simulink model "Md61Md62CalibSet"  (R2018b)
settings: Solver=FixedStepDiscrete  StartTime=0.0  StopTime=10.0  FixedStep=0.01  RelTol=1e-3
undefined symbols (not defined in the file or in its folder): KeSMSuFirstRwStBackPosDelta_Val, KeSMSuFirstRwStCushFoldPosDelta_Val, KeSMSuFirstRwStFwdBkwdPosDelta_Val, KeSMSuThrdRwCushFoldPosDelta_Val, KeSMSwAcsMd30PassStBkReclnUpwdDnwdPos1_Val, KeSMSwAcsMd30PassStBkReclnUpwdDnwdPos1Max_Val, KeSMSwAcsMd30PassStBkReclnUpwdDnwdPos1Min_Val, KeSMSwAcsMd30PassStFldUpwdDnwdPos1_Val, KeSMSwAcsMd30PassStFrwdBkwdPos1_Val, KeSMSwAcsMd30PassStFrwdBkwdPos1Max_Val, KeSMSwAcsMd30PassStFrwdBkwdPos1Min_Val, KeSMSwSeatBkLimitPos_Val, KeSMSwSeatBkLimitPosDelt_Val
libraries: StIsPosChkLib x2
(part 3 of 5)

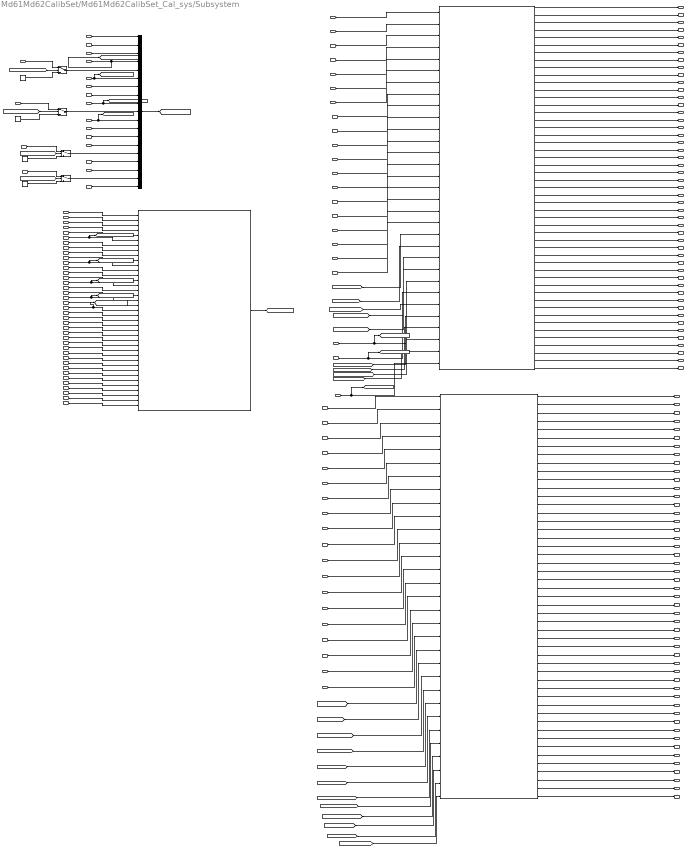
== system Md61Md62CalibSet/Md61Md62CalibSet_Cal_sys/Subsystem ==
  EepMd61PassStBkReclnTrgtPos_Val_read : Inport
  EepMd61PassStCshnFldTrgtPos_Val_read : Inport  Port=2
  EepMd61PassStFwdBkwdTrgtPos_Val_read : Inport  Port=3
  EepMd61SecRwLtStBkReclnTrgtPos_Val_read : Inport  Port=4
  EepMd61SecRwLtStCushFrntTrgtPos_Val_read : Inport  Port=5
  EepMd61SecRwLtStFwdBkwdTrgtPos_Val_read : Inport  Port=6
  EepMd61SecRwLtStLgrstInwdOtwdTrgtPos_Val_read : Inport  Port=7
  EepMd61SecRwLtStLgrstUpwdDnwdTrgtPos_Val_read : Inport  Port=8
  EepMd61SecRwRtStBkReclnTrgtPos_Val_read : Inport  Port=9
  EepMd61SecRwRtStCushFrntTrgtPos_Val_read : Inport  Port=10
  EepMd61SecRwRtStFwdBkwdTrgtPos_Val_read : Inport  Port=11
  EepMd61SecRwRtStLgrstInwdOtwdTrgtPos_Val_read : Inport  Port=12
  EepMd61SecRwRtStLgrstUpwdDnwdTrgtPos_Val_read : Inport  Port=13
  EepMd61ThdRwLtStBkReclnTrgtPos_Val_read : Inport  Port=14
  EepMd61ThdRwLtStCshnFldTrgtPos_Val_read : Inport  Port=15
  EepMd61ThdRwLtStFwdBkwdTrgtPos_Val_read : Inport  Port=16
  EepMd61ThdRwRtStBkReclnTrgtPos_Val_read : Inport  Port=17
  EepMd61ThdRwRtStCshnFldTrgtPos_Val_read : Inport  Port=18
  EepMd61ThdRwRtStFwdBkwdTrgtPos_Val_read : Inport  Port=19
  EepMd62PassStBkReclnTrgtPos_Val_read : Inport  Port=20
  EepMd62PassStCshnFldTrgtPos_Val_read : Inport  Port=21
  EepMd62PassStFwdBkwdTrgtPos_Val_read : Inport  Port=22
  EepMd62SecRwLtStBkReclnTrgtPos_Val_read : Inport  Port=23
  EepMd62SecRwLtStCushFrntTrgtPos_Val_read : Inport  Port=24
  EepMd62SecRwLtStFwdBkwdTrgtPos_Val_read : Inport  Port=25
  EepMd62SecRwLtStLgrstInwdOtwdTrgtPos_Val_read : Inport  Port=26
  EepMd62SecRwLtStLgrstUpwdDnwdTrgtPos_Val_read : Inport  Port=27
  EepMd62SecRwRtStBkReclnTrgtPos_Val_read : Inport  Port=28
  EepMd62SecRwRtStCushFrntTrgtPos_Val_read : Inport  Port=29
  EepMd62SecRwRtStFwdBkwdTrgtPos_Val_read : Inport  Port=30
  EepMd62SecRwRtStLgrstInwdOtwdTrgtPos_Val_read : Inport  Port=31
  EepMd62SecRwRtStLgrstUpwdDnwdTrgtPos_Val_read : Inport  Port=32
  EepMd62ThdRwLtStBkReclnTrgtPos_Val_read : Inport  Port=33
  EepMd62ThdRwLtStCshnFldTrgtPos_Val_read : Inport  Port=34
  EepMd62ThdRwLtStFwdBkwdTrgtPos_Val_read : Inport  Port=35
  EepMd62ThdRwRtStBkReclnTrgtPos_Val_read : Inport  Port=36
  EepMd62ThdRwRtStCshnFldTrgtPos_Val_read : Inport  Port=37
  EepMd62ThdRwRtStFwdBkwdTrgtPos_Val_read : Inport  Port=38
  IfVeSMSbPassStBkReclnUpwdDnwdMovConfig_Val_read : Inport  Port=39
  IfVeSMSbPassStFldUpwdDnwdMovConfig_Val_read : Inport  Port=40
  IfVeSMSbPassStFrwdBkwdMovConfig_Val_read : Inport  Port=41
  IfVeSMSbSecRwLtSLgrstExpdMovConfig_Val_read : Inport  Port=42
  IfVeSMSbSecRwLtStBkReclnUpwdDnwdMovConfig_Val_read : Inport  Port=43
  IfVeSMSbSecRwLtStCshnFrntUpwdDnwdMovConfig_Val_read : Inport  Port=44
  IfVeSMSbSecRwLtStFrwdBkwdMovConfig_Val_read : Inport  Port=45
  IfVeSMSbSecRwLtStLgrstUpwdMovConfig_Val_read : Inport  Port=46
  IfVeSMSbSecRwRtSLgrstExpdMovConfig_Val_read : Inport  Port=47
  IfVeSMSbSecRwRtStBkReclnUpwdDnwdMovConfig_Val_read : Inport  Port=48
  IfVeSMSbSecRwRtStCshnFrntUpwdDnwdMovConfig_Val_read : Inport  Port=49
  IfVeSMSbSecRwRtStFrwdBkwdMovConfig_Val_read : Inport  Port=50
  IfVeSMSbSecRwRtStLgrstUpwdMovConfig_Val_read : Inport  Port=51
  IfVeSMSbThdRwLtStBkReclnUpwdDnwdMovConfig_Val_read : Inport  Port=52
  IfVeSMSbThdRwLtStCshnFldUpwdDnwdMovConfig_Val_read : Inport  Port=53
  IfVeSMSbThdRwLtStFrwdBkwdMovConfig_Val_read : Inport  Port=54
  IfVeSMSbThdRwRtStBkReclnUpwdDnwdMovConfig_Val_read : Inport  Port=55
  IfVeSMSbThdRwRtStCshnFldUpwdDnwdMovConfig_Val_read : Inport  Port=56
  IfVeSMSbThdRwRtStFrwdBkwdMovConfig_Val_read : Inport  Port=57
  IfVeSMSuPassStBkReclnUpwdDnwdPos_Val_read : Inport  Port=58
  IfVeSMSuPassStBkReclnUpwdDnwdPosV_Val_read : Inport  Port=59
  IfVeSMSuPassStFldUpwdDnwdPos_Val_read : Inport  Port=60
  IfVeSMSuPassStFldUpwdDnwdPosV_Val_read : Inport  Port=61
  IfVeSMSuPassStFrwdBkwdPos_Val_read : Inport  Port=62
  IfVeSMSuPassStFrwdBkwdPosV_Val_read : Inport  Port=63
  IfVeSMSuSecRwLtStBkReclnUpwdDnwdPos_Val_read : Inport  Port=64
  IfVeSMSuSecRwLtStBkReclnUpwdDnwdPosV_Val_read : Inport  Port=65
  IfVeSMSuSecRwLtStFrwdBkwdPos_Val_read : Inport  Port=66
  IfVeSMSuSecRwLtStFrwdBkwdPosV_Val_read : Inport  Port=67
  IfVeSMSuSecRwLtStLgrstOtwdInwdPos_Val_read : Inport  Port=68
  IfVeSMSuSecRwLtStLgrstOtwdInwdPosV_Val_read : Inport  Port=69
  IfVeSMSuSecRwLtStLgrstUpwdDnwdPos_Val_read : Inport  Port=70
  IfVeSMSuSecRwLtStLgrstUpwdDnwdPosV_Val_read : Inport  Port=71
  IfVeSMSuSecRwLtStZeroPos_Val_read : Inport  Port=72
  IfVeSMSuSecRwLtStZeroPosV_Val_read : Inport  Port=73
  IfVeSMSuSecRwRtStBkReclnUpwdDnwdPos_Val_read : Inport  Port=74
  IfVeSMSuSecRwRtStBkReclnUpwdDnwdPosV_Val_read : Inport  Port=75
  IfVeSMSuSecRwRtStFrwdBkwdPos_Val_read : Inport  Port=76
  IfVeSMSuSecRwRtStFrwdBkwdPosV_Val_read : Inport  Port=77
  IfVeSMSuSecRwRtStLgrstOtwdInwdPos_Val_read : Inport  Port=78
  IfVeSMSuSecRwRtStLgrstOtwdInwdPosV_Val_read : Inport  Port=79
  IfVeSMSuSecRwRtStLgrstUpwdDnwdPos_Val_read : Inport  Port=80
  IfVeSMSuSecRwRtStLgrstUpwdDnwdPosV_Val_read : Inport  Port=81
  IfVeSMSuSecRwRtStZeroPos_Val_read : Inport  Port=82
  IfVeSMSuSecRwRtStZeroPosV_Val_read : Inport  Port=83
  IfVeSMSuThdRwLtStBkReclnUpwdDnwdPos_Val_read : Inport  Port=84
  IfVeSMSuThdRwLtStBkReclnUpwdDnwdPosV_Val_read : Inport  Port=85
  IfVeSMSuThdRwLtStCshnFldUpwdDnwdPos_Val_read : Inport  Port=86
  IfVeSMSuThdRwLtStCshnFldUpwdDnwdPosV_Val_read : Inport  Port=87
  IfVeSMSuThdRwLtStFrwdBkwdPos_Val_read : Inport  Port=88
  IfVeSMSuThdRwLtStFrwdBkwdPosV_Val_read : Inport  Port=89
  IfVeSMSuThdRwRtStBkReclnUpwdDnwdPos_Val_read : Inport  Port=90
  IfVeSMSuThdRwRtStBkReclnUpwdDnwdPosV_Val_read : Inport  Port=91
  IfVeSMSuThdRwRtStCshnFldUpwdDnwdPos_Val_read : Inport  Port=92
  IfVeSMSuThdRwRtStCshnFldUpwdDnwdPosV_Val_read : Inport  Port=93
  IfVeSMSuThdRwRtStFrwdBkwdPos_Val_read : Inport  Port=94
  IfVeSMSuThdRwRtStFrwdBkwdPosV_Val_read : Inport  Port=95
  StPassCmprtRestMdMemVirtCtrlReqMdadjust_Val_read : Inport  Port=96
  KeSMSwSeatBkLimitPos_Val : Inport  Port=97
  KeSMSwSeatBkLimitPosDelt_Val : Inport  Port=98
  modestate32_Val_read : Inport  Port=99
  Constant{,1..3} (4 alike) : Constant  Value=4095  OutDataTypeStr=uint16
  Md61Calib : Subsystem
  Md62Calib : Subsystem
  MemReqChk : Subsystem
  Mux : Mux  Inputs=19
  Switch{,1..3} (4 alike) : Switch  Criteria=u2 > Threshold
  Md61PassStBkReclnTrgtPos_Val_write : Outport
      settings: EnsureOutportIsVirtual=on
  Md61PassStBkReclnTrgtPosCalib_TrgtPosArray_write : Outport  Port=2
      settings: EnsureOutportIsVirtual=on
  Md61PassStCshnFldTrgtPosCalib_TrgtPosArray_write : Outport  Port=3
      settings: EnsureOutportIsVirtual=on
  Md61PassStFwdBkwdTrgtPosCalib_TrgtPosArray_write : Outport  Port=4
      settings: EnsureOutportIsVirtual=on
  Md61SecRwLtStBkReclnTrgtPosCalib_TrgtPosArray_write : Outport  Port=5
      settings: EnsureOutportIsVirtual=on
  Md61SecRwLtStCushFrntTrgtPosCalib_TrgtPosArray_write : Outport  Port=6
      settings: EnsureOutportIsVirtual=on
  Md61SecRwLtStFwdBkwdCalib_TrgtPosArray_write : Outport  Port=7
      settings: EnsureOutportIsVirtual=on
  Md61SecRwLtStLgrstInwdOtwdTrgtPosCalib_TrgtPosArray_write : Outport  Port=8
      settings: EnsureOutportIsVirtual=on
  Md61SecRwLtStLgrstUpwdDnwdTrgtPosCalib_TrgtPosArray_write : Outport  Port=9
      settings: EnsureOutportIsVirtual=on
  Md61ThdRwLtStBkReclnUpwdDnwdTrgtPosCalib_TrgtPosArray_write : Outport  Port=10
      settings: EnsureOutportIsVirtual=on
  Md61ThdRwLtStCshnFldUpwdDnwdTrgtPos_Val_write : Outport  Port=11
      settings: EnsureOutportIsVirtual=on
  Md61ThdRwLtStCshnFldUpwdDnwdTrgtPosCalib_TrgtPosArray_write : Outport  Port=12
      settings: EnsureOutportIsVirtual=on
  Md61ThdRwLtStFrwdBkwdPosTrgtPosCalib_TrgtPosArray_write : Outport  Port=13
      settings: EnsureOutportIsVirtual=on
  Md61ThdRwRtStCshnFldUpwdDnwdTrgtPos_Val_write : Outport  Port=14
      settings: EnsureOutportIsVirtual=on
  Md62PassStBkReclnTrgtPos_Val_write : Outport  Port=15
      settings: EnsureOutportIsVirtual=on
  Md62PassStBkReclnTrgtPosCalib_TrgtPosArray_write : Outport  Port=16
      settings: EnsureOutportIsVirtual=on
  Md62PassStCshnFldTrgtPosCalib_TrgtPosArray_write : Outport  Port=17
      settings: EnsureOutportIsVirtual=on
  Md62PassStFwdBkwdTrgtPosCalib_TrgtPosArray_write : Outport  Port=18
      settings: EnsureOutportIsVirtual=on
  Md62SecRwLtStBkReclnTrgtPosCalib_TrgtPosArray_write : Outport  Port=19
      settings: EnsureOutportIsVirtual=on
  Md62SecRwLtStCushFrntTrgtPosCalib_TrgtPosArray_write : Outport  Port=20
      settings: EnsureOutportIsVirtual=on
  Md62SecRwLtStFwdBkwdCalib_TrgtPosArray_write : Outport  Port=21
      settings: EnsureOutportIsVirtual=on
  Md62SecRwLtStLgrstInwdOtwdTrgtPosCalib_TrgtPosArray_write : Outport  Port=22
      settings: EnsureOutportIsVirtual=on
  Md62SecRwLtStLgrstUpwdDnwdTrgtPosCalib_TrgtPosArray_write : Outport  Port=23
      settings: EnsureOutportIsVirtual=on
  Md62ThdRwLtStBkReclnUpwdDnwdTrgtPosCalib_TrgtPosArray_write : Outport  Port=24
      settings: EnsureOutportIsVirtual=on
  Md62ThdRwLtStCshnFldUpwdDnwdTrgtPos_Val_write : Outport  Port=25
      settings: EnsureOutportIsVirtual=on
  Md62ThdRwLtStCshnFldUpwdDnwdTrgtPosCalib_TrgtPosArray_write : Outport  Port=26
      settings: EnsureOutportIsVirtual=on
  Md62ThdRwLtStFrwdBkwdPosTrgtPosCalib_TrgtPosArray_write : Outport  Port=27
      settings: EnsureOutportIsVirtual=on
  Md62ThdRwRtStCshnFldUpwdDnwdTrgtPos_Val_write : Outport  Port=28
      settings: EnsureOutportIsVirtual=on
  Md61SecRwRtStBkReclnTrgtPosCalib_TrgtPosArray_write : Outport  Port=29
      settings: EnsureOutportIsVirtual=on
  Md61SecRwRtStCushFrntTrgtPosCalib_TrgtPosArray_write : Outport  Port=30
      settings: EnsureOutportIsVirtual=on
  Md61SecRwRtStFwdBkwdCalib_TrgtPosArray_write : Outport  Port=31
      settings: EnsureOutportIsVirtual=on
  Md61SecRwRtStLgrstInwdOtwdTrgtPosCalib_TrgtPosArray_write : Outport  Port=32
      settings: EnsureOutportIsVirtual=on
  Md61SecRwRtStLgrstUpwdDnwdTrgtPosCalib_TrgtPosArray_write : Outport  Port=33
      settings: EnsureOutportIsVirtual=on
  Md61ThdRwRtStBkReclnUpwdDnwdTrgtPosCalib_TrgtPosArray_write : Outport  Port=34
      settings: EnsureOutportIsVirtual=on
  Md61ThdRwRtStCshnFldUpwdDnwdTrgtPosCalib_TrgtPosArray_write : Outport  Port=35
      settings: EnsureOutportIsVirtual=on
  Md61ThdRwRtStFrwdBkwdPosTrgtPosCalib_TrgtPosArray_write : Outport  Port=36
      settings: EnsureOutportIsVirtual=on
  Md62SecRwRtStBkReclnTrgtPosCalib_TrgtPosArray_write : Outport  Port=37
      settings: EnsureOutportIsVirtual=on
  Md62SecRwRtStCushFrntTrgtPosCalib_TrgtPosArray_write : Outport  Port=38
      settings: EnsureOutportIsVirtual=on
  Md62SecRwRtStFwdBkwdCalib_TrgtPosArray_write : Outport  Port=39
      settings: EnsureOutportIsVirtual=on
  Md62SecRwRtStLgrstInwdOtwdTrgtPosCalib_TrgtPosArray_write : Outport  Port=40
      settings: EnsureOutportIsVirtual=on
  Md62SecRwRtStLgrstUpwdDnwdTrgtPosCalib_TrgtPosArray_write : Outport  Port=41
      settings: EnsureOutportIsVirtual=on
  Md62ThdRwRtStBkReclnUpwdDnwdTrgtPosCalib_TrgtPosArray_write : Outport  Port=42
      settings: EnsureOutportIsVirtual=on
  Md62ThdRwRtStCshnFldUpwdDnwdTrgtPosCalib_TrgtPosArray_write : Outport  Port=43
      settings: EnsureOutportIsVirtual=on
  Md62ThdRwRtStFrwdBkwdPosTrgtPosCalib_TrgtPosArray_write : Outport  Port=44
      settings: EnsureOutportIsVirtual=on
  Md61PassStNeedFldOpn_Val_write : Outport  Port=45
      settings: EnsureOutportIsVirtual=on
  Md61PassStTrgtIsFld_Val_write : Outport  Port=46
      settings: EnsureOutportIsVirtual=on
  Md61ThdRwLtStNeedFldOpn_Val_write : Outport  Port=47
      settings: EnsureOutportIsVirtual=on
  Md61ThdRwLtStTrgtIsFld_Val_write : Outport  Port=48
      settings: EnsureOutportIsVirtual=on
  Md61ThdRwRtStNeedFldOpn_Val_write : Outport  Port=49
      settings: EnsureOutportIsVirtual=on
  Md61ThdRwRtStTrgtIsFld_Val_write : Outport  Port=50
      settings: EnsureOutportIsVirtual=on
  Md62PassStNeedFldOpn_Val_write : Outport  Port=51
      settings: EnsureOutportIsVirtual=on
  Md62PassStTrgtIsFld_Val_write : Outport  Port=52
      settings: EnsureOutportIsVirtual=on
  Md62ThdRwLtStNeedFldOpn_Val_write : Outport  Port=53
      settings: EnsureOutportIsVirtual=on
  Md62ThdRwLtStTrgtIsFld_Val_write : Outport  Port=54
      settings: EnsureOutportIsVirtual=on
  Md62ThdRwRtStNeedFldOpn_Val_write : Outport  Port=55
      settings: EnsureOutportIsVirtual=on
  Md62ThdRwRtStTrgtIsFld_Val_write : Outport  Port=56
      settings: EnsureOutportIsVirtual=on
  EepMd61PassStBkReclnTrgtPos_S_Val_write : Outport  Port=57
      settings: EnsureOutportIsVirtual=on
  EepMd61PassStCshnFldTrgtPos_S_Val_write : Outport  Port=58
      settings: EnsureOutportIsVirtual=on
  EepMd61PassStFwdBkwdTrgtPos_S_Val_write : Outport  Port=59
      settings: EnsureOutportIsVirtual=on
  EepMd61SecRwLtStBkReclnTrgtPos_S_Val_write : Outport  Port=60
      settings: EnsureOutportIsVirtual=on
  EepMd61SecRwLtStCushFrntTrgtPos_S_Val_write : Outport  Port=61
      settings: EnsureOutportIsVirtual=on
  EepMd61SecRwLtStFwdBkwdTrgtPos_S_Val_write : Outport  Port=62
      settings: EnsureOutportIsVirtual=on
  EepMd61SecRwLtStLgrstInwdOtwdTrgtPos_S_Val_write : Outport  Port=63
      settings: EnsureOutportIsVirtual=on
  EepMd61SecRwLtStLgrstUpwdDnwdTrgtPos_S_Val_write : Outport  Port=64
      settings: EnsureOutportIsVirtual=on
  EepMd61SecRwRtStBkReclnTrgtPos_S_Val_write : Outport  Port=65
      settings: EnsureOutportIsVirtual=on
  EepMd61SecRwRtStCushFrntTrgtPos_S_Val_write : Outport  Port=66
      settings: EnsureOutportIsVirtual=on
  EepMd61SecRwRtStFwdBkwdTrgtPos_S_Val_write : Outport  Port=67
      settings: EnsureOutportIsVirtual=on
  EepMd61SecRwRtStLgrstInwdOtwdTrgtPos_S_Val_write : Outport  Port=68
      settings: EnsureOutportIsVirtual=on
  EepMd61SecRwRtStLgrstUpwdDnwdTrgtPos_S_Val_write : Outport  Port=69
      settings: EnsureOutportIsVirtual=on
  EepMd61ThdRwLtStBkReclnTrgtPos_S_Val_write : Outport  Port=70
      settings: EnsureOutportIsVirtual=on
  EepMd61ThdRwLtStCshnFldTrgtPos_S_Val_write : Outport  Port=71
      settings: EnsureOutportIsVirtual=on
  EepMd61ThdRwLtStFwdBkwdTrgtPos_S_Val_write : Outport  Port=72
      settings: EnsureOutportIsVirtual=on
  EepMd61ThdRwRtStBkReclnTrgtPos_S_Val_write : Outport  Port=73
      settings: EnsureOutportIsVirtual=on
  EepMd61ThdRwRtStCshnFldTrgtPos_S_Val_write : Outport  Port=74
      settings: EnsureOutportIsVirtual=on
  EepMd61ThdRwRtStFwdBkwdTrgtPos_S_Val_write : Outport  Port=75
      settings: EnsureOutportIsVirtual=on
  EepMd62PassStBkReclnTrgtPos_S_Val_write : Outport  Port=76
      settings: EnsureOutportIsVirtual=on
  EepMd62PassStCshnFldTrgtPos_S_Val_write : Outport  Port=77
      settings: EnsureOutportIsVirtual=on
  EepMd62PassStFwdBkwdTrgtPos_S_Val_write : Outport  Port=78
      settings: EnsureOutportIsVirtual=on
  EepMd62SecRwLtStBkReclnTrgtPos_S_Val_write : Outport  Port=79
      settings: EnsureOutportIsVirtual=on
  EepMd62SecRwLtStCushFrntTrgtPos_S_Val_write : Outport  Port=80
      settings: EnsureOutportIsVirtual=on
  EepMd62SecRwLtStFwdBkwdTrgtPos_S_Val_write : Outport  Port=81
      settings: EnsureOutportIsVirtual=on
  EepMd62SecRwLtStLgrstInwdOtwdTrgtPos_S_Val_write : Outport  Port=82
      settings: EnsureOutportIsVirtual=on
  EepMd62SecRwLtStLgrstUpwdDnwdTrgtPos_S_Val_write : Outport  Port=83
      settings: EnsureOutportIsVirtual=on
  EepMd62SecRwRtStBkReclnTrgtPos_S_Val_write : Outport  Port=84
      settings: EnsureOutportIsVirtual=on
  EepMd62SecRwRtStCushFrntTrgtPos_S_Val_write : Outport  Port=85
      settings: EnsureOutportIsVirtual=on
  EepMd62SecRwRtStFwdBkwdTrgtPos_S_Val_write : Outport  Port=86
      settings: EnsureOutportIsVirtual=on
  EepMd62SecRwRtStLgrstInwdOtwdTrgtPos_S_Val_write : Outport  Port=87
      settings: EnsureOutportIsVirtual=on
  EepMd62SecRwRtStLgrstUpwdDnwdTrgtPos_S_Val_write : Outport  Port=88
      settings: EnsureOutportIsVirtual=on
  EepMd62ThdRwLtStBkReclnTrgtPos_S_Val_write : Outport  Port=89
      settings: EnsureOutportIsVirtual=on
  EepMd62ThdRwLtStCshnFldTrgtPos_S_Val_write : Outport  Port=90
      settings: EnsureOutportIsVirtual=on
  EepMd62ThdRwLtStFwdBkwdTrgtPos_S_Val_write : Outport  Port=91
      settings: EnsureOutportIsVirtual=on
  EepMd62ThdRwRtStBkReclnTrgtPos_S_Val_write : Outport  Port=92
      settings: EnsureOutportIsVirtual=on
  EepMd62ThdRwRtStCshnFldTrgtPos_S_Val_write : Outport  Port=93
      settings: EnsureOutportIsVirtual=on
  EepMd62ThdRwRtStFwdBkwdTrgtPos_S_Val_write : Outport  Port=94
      settings: EnsureOutportIsVirtual=on
  Md61MemReq_Val_write : Outport  Port=95
      settings: EnsureOutportIsVirtual=on
  Md62MemReq_Val_write : Outport  Port=96
      settings: EnsureOutportIsVirtual=on
  Md61NotMem_Val_write : Outport  Port=97
      settings: EnsureOutportIsVirtual=on
  Md62NotMem_Val_write : Outport  Port=98
      settings: EnsureOutportIsVirtual=on
  wires:
  [MemReq] -> Md61Calib/21(MemReq)
  EepMd61PassStCshnFldTrgtPos_Val_read/1 -> Md61Calib/2(EepMd61PassStCshnFldTrgtPos_Val_read)
  EepMd61PassStBkReclnTrgtPos_Val_read/1 -> Md61Calib/1(EepMd61PassStBkReclnTrgtPos_Val_read)
  EepMd61PassStFwdBkwdTrgtPos_Val_read/1 -> Md61Calib/3(EepMd61PassStFwdBkwdTrgtPos_Val_read)
  EepMd61SecRwLtStBkReclnTrgtPos_Val_read/1 -> Md61Calib/4(EepMd61SecRwLtStBkReclnTrgtPos_Val_read)
  EepMd61SecRwLtStCushFrntTrgtPos_Val_read/1 -> Md61Calib/5(EepMd61SecRwLtStCushFrntTrgtPos_Val_read)
  EepMd61SecRwLtStFwdBkwdTrgtPos_Val_read/1 -> Md61Calib/6(EepMd61SecRwLtStFwdBkwdTrgtPos_Val_read)
  EepMd61SecRwLtStLgrstInwdOtwdTrgtPos_Val_read/1 -> Md61Calib/7(EepMd61SecRwLtStLgrstInwdOtwdTrgtPos_Val_read)
  EepMd61SecRwLtStLgrstUpwdDnwdTrgtPos_Val_read/1 -> Md61Calib/8(EepMd61SecRwLtStLgrstUpwdDnwdTrgtPos_Val_read)
  EepMd61SecRwRtStBkReclnTrgtPos_Val_read/1 -> Md61Calib/9(EepMd61SecRwRtStBkReclnTrgtPos_Val_read)
  EepMd61SecRwRtStCushFrntTrgtPos_Val_read/1 -> Md61Calib/10(EepMd61SecRwRtStCushFrntTrgtPos_Val_read)
  EepMd61SecRwRtStFwdBkwdTrgtPos_Val_read/1 -> Md61Calib/11(EepMd61SecRwRtStFwdBkwdTrgtPos_Val_read)
  EepMd61SecRwRtStLgrstInwdOtwdTrgtPos_Val_read/1 -> Md61Calib/12(EepMd61SecRwRtStLgrstInwdOtwdTrgtPos_Val_read)
  EepMd61SecRwRtStLgrstUpwdDnwdTrgtPos_Val_read/1 -> Md61Calib/13(EepMd61SecRwRtStLgrstUpwdDnwdTrgtPos_Val_read)
  EepMd61ThdRwLtStBkReclnTrgtPos_Val_read/1 -> Md61Calib/14(EepMd61ThdRwLtStBkReclnTrgtPos_Val_read)
  EepMd61ThdRwLtStCshnFldTrgtPos_Val_read/1 -> Md61Calib/15(EepMd61ThdRwLtStCshnFldTrgtPos_Val_read)
  EepMd61ThdRwLtStFwdBkwdTrgtPos_Val_read/1 -> Md61Calib/16(EepMd61ThdRwLtStFwdBkwdTrgtPos_Val_read)
  EepMd61ThdRwRtStBkReclnTrgtPos_Val_read/1 -> Md61Calib/17(EepMd61ThdRwRtStBkReclnTrgtPos_Val_read)
  EepMd61ThdRwRtStCshnFldTrgtPos_Val_read/1 -> Md61Calib/18(EepMd61ThdRwRtStCshnFldTrgtPos_Val_read)
  EepMd61ThdRwRtStFwdBkwdTrgtPos_Val_read/1 -> Md61Calib/19(EepMd61ThdRwRtStFwdBkwdTrgtPos_Val_read)
  IfVeSMSbPassStBkReclnUpwdDnwdMovConfig_Val_read/1 -> MemReqChk/1(IfVeSMSbPassStBkReclnUpwdDnwdMovConfig_Val_read)
  IfVeSMSbPassStFldUpwdDnwdMovConfig_Val_read/1 -> MemReqChk/2(IfVeSMSbPassStFldUpwdDnwdMovConfig_Val_read)
  IfVeSMSbPassStFrwdBkwdMovConfig_Val_read/1 -> MemReqChk/3(IfVeSMSbPassStFrwdBkwdMovConfig_Val_read)
  IfVeSMSbSecRwLtSLgrstExpdMovConfig_Val_read/1 -> MemReqChk/4(IfVeSMSbSecRwLtSLgrstExpdMovConfig_Val_read)
  IfVeSMSbSecRwLtStBkReclnUpwdDnwdMovConfig_Val_read/1 -> MemReqChk/5(IfVeSMSbSecRwLtStBkReclnUpwdDnwdMovConfig_Val_read)
  IfVeSMSbSecRwLtStCshnFrntUpwdDnwdMovConfig_Val_read/1 -> [SecRwLtStCshnFrntUpwdDnwdMovConfig], MemReqChk/6(IfVeSMSbSecRwLtStCshnFrntUpwdDnwdMovConfig_Val_read)
  IfVeSMSbSecRwLtStFrwdBkwdMovConfig_Val_read/1 -> MemReqChk/7(IfVeSMSbSecRwLtStFrwdBkwdMovConfig_Val_read)
  IfVeSMSbSecRwLtStLgrstUpwdMovConfig_Val_read/1 -> MemReqChk/8(IfVeSMSbSecRwLtStLgrstUpwdMovConfig_Val_read)
  IfVeSMSbSecRwRtSLgrstExpdMovConfig_Val_read/1 -> MemReqChk/9(IfVeSMSbSecRwRtSLgrstExpdMovConfig_Val_read)
  IfVeSMSbSecRwRtStBkReclnUpwdDnwdMovConfig_Val_read/1 -> MemReqChk/10(IfVeSMSbSecRwRtStBkReclnUpwdDnwdMovConfig_Val_read)
  IfVeSMSbSecRwRtStCshnFrntUpwdDnwdMovConfig_Val_read/1 -> MemReqChk/11(IfVeSMSbSecRwRtStCshnFrntUpwdDnwdMovConfig_Val_read), [SecRwRtStCshnFrntUpwdDnwdMovConfig]
  IfVeSMSbSecRwRtStFrwdBkwdMovConfig_Val_read/1 -> MemReqChk/12(IfVeSMSbSecRwRtStFrwdBkwdMovConfig_Val_read)
  IfVeSMSbSecRwRtStLgrstUpwdMovConfig_Val_read/1 -> MemReqChk/13(IfVeSMSbSecRwRtStLgrstUpwdMovConfig_Val_read)
  IfVeSMSbThdRwLtStBkReclnUpwdDnwdMovConfig_Val_read/1 -> MemReqChk/14(IfVeSMSbThdRwLtStBkReclnUpwdDnwdMovConfig_Val_read)
  IfVeSMSbThdRwLtStCshnFldUpwdDnwdMovConfig_Val_read/1 -> [ThdRwLtStCshnFldUpwdDnwdMovConfig], MemReqChk/15(IfVeSMSbThdRwLtStCshnFldUpwdDnwdMovConfig_Val_read)
  IfVeSMSbThdRwLtStFrwdBkwdMovConfig_Val_read/1 -> MemReqChk/16(IfVeSMSbThdRwLtStFrwdBkwdMovConfig_Val_read)
  IfVeSMSbThdRwRtStBkReclnUpwdDnwdMovConfig_Val_read/1 -> MemReqChk/17(IfVeSMSbThdRwRtStBkReclnUpwdDnwdMovConfig_Val_read)
  IfVeSMSbThdRwRtStCshnFldUpwdDnwdMovConfig_Val_read/1 -> [ThdRwRtStCshnFldUpwdDnwdMovConfig], MemReqChk/18(IfVeSMSbThdRwRtStCshnFldUpwdDnwdMovConfig_Val_read)
  IfVeSMSbThdRwRtStFrwdBkwdMovConfig_Val_read/1 -> MemReqChk/19(IfVeSMSbThdRwRtStFrwdBkwdMovConfig_Val_read)
  IfVeSMSuPassStBkReclnUpwdDnwdPosV_Val_read/1 -> [IfVeSMSuPassStBkReclnUpwdDnwdPosV], MemReqChk/20(IfVeSMSuPassStBkReclnUpwdDnwdPosV_Val_read)
  IfVeSMSuPassStFldUpwdDnwdPosV_Val_read/1 -> MemReqChk/21(IfVeSMSuPassStFldUpwdDnwdPosV_Val_read)
  IfVeSMSuPassStFrwdBkwdPosV_Val_read/1 -> MemReqChk/22(IfVeSMSuPassStFrwdBkwdPosV_Val_read)
  IfVeSMSuSecRwLtStBkReclnUpwdDnwdPosV_Val_read/1 -> MemReqChk/23(IfVeSMSuSecRwLtStBkReclnUpwdDnwdPosV_Val_read)
  IfVeSMSuSecRwLtStFrwdBkwdPosV_Val_read/1 -> MemReqChk/24(IfVeSMSuSecRwLtStFrwdBkwdPosV_Val_read)
  IfVeSMSuSecRwLtStLgrstOtwdInwdPosV_Val_read/1 -> MemReqChk/25(IfVeSMSuSecRwLtStLgrstOtwdInwdPosV_Val_read)
  IfVeSMSuSecRwLtStLgrstUpwdDnwdPosV_Val_read/1 -> MemReqChk/26(IfVeSMSuSecRwLtStLgrstUpwdDnwdPosV_Val_read)
  IfVeSMSuSecRwLtStZeroPosV_Val_read/1 -> MemReqChk/27(IfVeSMSuSecRwLtStZeroPosV_Val_read)
  IfVeSMSuSecRwRtStBkReclnUpwdDnwdPosV_Val_read/1 -> MemReqChk/28(IfVeSMSuSecRwRtStBkReclnUpwdDnwdPosV_Val_read)
  IfVeSMSuSecRwRtStFrwdBkwdPosV_Val_read/1 -> MemReqChk/29(IfVeSMSuSecRwRtStFrwdBkwdPosV_Val_read)
  IfVeSMSuSecRwRtStLgrstOtwdInwdPosV_Val_read/1 -> MemReqChk/30(IfVeSMSuSecRwRtStLgrstOtwdInwdPosV_Val_read)
  IfVeSMSuSecRwRtStLgrstUpwdDnwdPosV_Val_read/1 -> MemReqChk/31(IfVeSMSuSecRwRtStLgrstUpwdDnwdPosV_Val_read)
  IfVeSMSuSecRwRtStZeroPosV_Val_read/1 -> MemReqChk/32(IfVeSMSuSecRwRtStZeroPosV_Val_read)
  IfVeSMSuThdRwLtStBkReclnUpwdDnwdPosV_Val_read/1 -> MemReqChk/33(IfVeSMSuThdRwLtStBkReclnUpwdDnwdPosV_Val_read)
  IfVeSMSuThdRwLtStCshnFldUpwdDnwdPosV_Val_read/1 -> MemReqChk/34(IfVeSMSuThdRwLtStCshnFldUpwdDnwdPosV_Val_read)
  IfVeSMSuThdRwLtStFrwdBkwdPosV_Val_read/1 -> MemReqChk/35(IfVeSMSuThdRwLtStFrwdBkwdPosV_Val_read)
  IfVeSMSuThdRwRtStBkReclnUpwdDnwdPosV_Val_read/1 -> MemReqChk/36(IfVeSMSuThdRwRtStBkReclnUpwdDnwdPosV_Val_read)
  IfVeSMSuThdRwRtStCshnFldUpwdDnwdPosV_Val_read/1 -> MemReqChk/37(IfVeSMSuThdRwRtStCshnFldUpwdDnwdPosV_Val_read)
  IfVeSMSuThdRwRtStFrwdBkwdPosV_Val_read/1 -> MemReqChk/38(IfVeSMSuThdRwRtStFrwdBkwdPosV_Val_read)
  StPassCmprtRestMdMemVirtCtrlReqMdadjust_Val_read/1 -> MemReqChk/39(StPassCmprtRestMdMemVirtCtrlReqMdadjust_Val_read)
  IfVeSMSuPassStBkReclnUpwdDnwdPos_Val_read/1 -> Mux/1
  IfVeSMSuPassStFldUpwdDnwdPos_Val_read/1 -> Mux/2
  IfVeSMSuPassStFrwdBkwdPos_Val_read/1 -> Mux/3
  IfVeSMSuSecRwLtStBkReclnUpwdDnwdPos_Val_read/1 -> Mux/4, [IfVeSMSuSecRwLtStBkReclnUpwdDnwdPos]
  IfVeSMSuSecRwRtStBkReclnUpwdDnwdPos_Val_read/1 -> [IfVeSMSuSecRwRtStBkReclnUpwdDnwdPos], Mux/9
  IfVeSMSuThdRwLtStBkReclnUpwdDnwdPos_Val_read/1 -> Mux/14
  IfVeSMSuThdRwLtStFrwdBkwdPos_Val_read/1 -> Mux/16
  IfVeSMSuThdRwRtStBkReclnUpwdDnwdPos_Val_read/1 -> Mux/17
  IfVeSMSuThdRwRtStFrwdBkwdPos_Val_read/1 -> Mux/19
  IfVeSMSuSecRwLtStFrwdBkwdPos_Val_read/1 -> [IfVeSMSuSecRwLtStFrwdBkwdPos], Mux/6
  IfVeSMSuSecRwLtStLgrstOtwdInwdPos_Val_read/1 -> Mux/7
  IfVeSMSuSecRwLtStLgrstUpwdDnwdPos_Val_read/1 -> Mux/8
  IfVeSMSuSecRwRtStFrwdBkwdPos_Val_read/1 -> [IfVeSMSuSecRwRtStFrwdBkwdPos], Mux/11
  IfVeSMSuSecRwRtStLgrstOtwdInwdPos_Val_read/1 -> Mux/12
  IfVeSMSuSecRwRtStLgrstUpwdDnwdPos_Val_read/1 -> Mux/13
  Mux/1 -> [CurrentPosArray]
  [CurrentPosArray] -> Md61Calib/20(CurrentPosArray)
  MemReqChk/1(MemReq) -> [MemReq]
  Md61Calib/2(Md61PassStBkReclnTrgtPosCalib_TrgtPosArray_write) -> Md61PassStBkReclnTrgtPosCalib_TrgtPosArray_write/1
  Md61Calib/3(Md61PassStCshnFldTrgtPosCalib_TrgtPosArray_write) -> Md61PassStCshnFldTrgtPosCalib_TrgtPosArray_write/1
  Md61Calib/1(Md61PassStBkReclnTrgtPos_Val_write) -> Md61PassStBkReclnTrgtPos_Val_write/1
  Md61Calib/4(Md61PassStFwdBkwdTrgtPosCalib_TrgtPosArray_write) -> Md61PassStFwdBkwdTrgtPosCalib_TrgtPosArray_write/1
  Md61Calib/5(Md61SecRwLtStBkReclnTrgtPosCalib_TrgtPosArray_write) -> Md61SecRwLtStBkReclnTrgtPosCalib_TrgtPosArray_write/1
  Md61Calib/6(Md61SecRwLtStCushFrntTrgtPosCalib_TrgtPosArray_write) -> Md61SecRwLtStCushFrntTrgtPosCalib_TrgtPosArray_write/1
  Md61Calib/7(Md61SecRwLtStFwdBkwdCalib_TrgtPosArray_write) -> Md61SecRwLtStFwdBkwdCalib_TrgtPosArray_write/1
  Md61Calib/8(Md61SecRwLtStLgrstInwdOtwdTrgtPosCalib_TrgtPosArray_write) -> Md61SecRwLtStLgrstInwdOtwdTrgtPosCalib_TrgtPosArray_write/1
  Md61Calib/9(Md61SecRwLtStLgrstUpwdDnwdTrgtPosCalib_TrgtPosArray_write) -> Md61SecRwLtStLgrstUpwdDnwdTrgtPosCalib_TrgtPosArray_write/1
  Md61Calib/10(Md61ThdRwLtStBkReclnUpwdDnwdTrgtPosCalib_TrgtPosArray_write) -> Md61ThdRwLtStBkReclnUpwdDnwdTrgtPosCalib_TrgtPosArray_write/1
  Md61Calib/11(Md61ThdRwLtStCshnFldUpwdDnwdTrgtPos_Val_write) -> Md61ThdRwLtStCshnFldUpwdDnwdTrgtPos_Val_write/1
  Md61Calib/12(Md61ThdRwLtStCshnFldUpwdDnwdTrgtPosCalib_TrgtPosArray_write) -> Md61ThdRwLtStCshnFldUpwdDnwdTrgtPosCalib_TrgtPosArray_write/1
  Md61Calib/13(Md61ThdRwLtStFrwdBkwdPosTrgtPosCalib_TrgtPosArray_write) -> Md61ThdRwLtStFrwdBkwdPosTrgtPosCalib_TrgtPosArray_write/1
  Md61Calib/14(Md61ThdRwRtStCshnFldUpwdDnwdTrgtPos_Val_write) -> Md61ThdRwRtStCshnFldUpwdDnwdTrgtPos_Val_write/1
  [ThdRwLtStCshnFldUpwdDnwdMovConfig] -> Switch/2
  IfVeSMSuThdRwLtStCshnFldUpwdDnwdPos_Val_read/1 -> Switch/1
  Switch/1 -> Mux/15
  Constant/1 -> Switch/3
  Switch1/1 -> Mux/18
  [ThdRwRtStCshnFldUpwdDnwdMovConfig] -> Switch1/2
  IfVeSMSuThdRwRtStCshnFldUpwdDnwdPos_Val_read/1 -> Switch1/1
  Constant1/1 -> Switch1/3
  Switch2/1 -> Mux/10
  [SecRwRtStCshnFrntUpwdDnwdMovConfig] -> Switch2/2
  IfVeSMSuSecRwRtStZeroPos_Val_read/1 -> Switch2/1
  Constant2/1 -> Switch2/3
  Switch3/1 -> Mux/5
  [SecRwLtStCshnFrntUpwdDnwdMovConfig] -> Switch3/2
  IfVeSMSuSecRwLtStZeroPos_Val_read/1 -> Switch3/1
  Constant3/1 -> Switch3/3
  EepMd62SecRwLtStFwdBkwdTrgtPos_Val_read/1 -> Md62Calib/6(EepMd62SecRwLtStFwdBkwdTrgtPos_Val_read)
  EepMd62SecRwLtStCushFrntTrgtPos_Val_read/1 -> Md62Calib/5(EepMd62SecRwLtStCushFrntTrgtPos_Val_read)
  EepMd62SecRwLtStLgrstInwdOtwdTrgtPos_Val_read/1 -> Md62Calib/7(EepMd62SecRwLtStLgrstInwdOtwdTrgtPos_Val_read)
  EepMd62SecRwLtStBkReclnTrgtPos_Val_read/1 -> Md62Calib/4(EepMd62SecRwLtStBkReclnTrgtPos_Val_read)
  EepMd62SecRwLtStLgrstUpwdDnwdTrgtPos_Val_read/1 -> Md62Calib/8(EepMd62SecRwLtStLgrstUpwdDnwdTrgtPos_Val_read)
  EepMd62PassStFwdBkwdTrgtPos_Val_read/1 -> Md62Calib/3(EepMd62PassStFwdBkwdTrgtPos_Val_read)
  EepMd62SecRwRtStBkReclnTrgtPos_Val_read/1 -> Md62Calib/9(EepMd62SecRwRtStBkReclnTrgtPos_Val_read)
  EepMd62PassStCshnFldTrgtPos_Val_read/1 -> Md62Calib/2(EepMd62PassStCshnFldTrgtPos_Val_read)
  EepMd62SecRwRtStCushFrntTrgtPos_Val_read/1 -> Md62Calib/10(EepMd62SecRwRtStCushFrntTrgtPos_Val_read)
  EepMd62PassStBkReclnTrgtPos_Val_read/1 -> Md62Calib/1(EepMd62PassStBkReclnTrgtPos_Val_read)
  EepMd62SecRwRtStFwdBkwdTrgtPos_Val_read/1 -> Md62Calib/11(EepMd62SecRwRtStFwdBkwdTrgtPos_Val_read)
  EepMd62SecRwRtStLgrstInwdOtwdTrgtPos_Val_read/1 -> Md62Calib/12(EepMd62SecRwRtStLgrstInwdOtwdTrgtPos_Val_read)
  EepMd62SecRwRtStLgrstUpwdDnwdTrgtPos_Val_read/1 -> Md62Calib/13(EepMd62SecRwRtStLgrstUpwdDnwdTrgtPos_Val_read)
  EepMd62ThdRwLtStBkReclnTrgtPos_Val_read/1 -> Md62Calib/14(EepMd62ThdRwLtStBkReclnTrgtPos_Val_read)
  EepMd62ThdRwLtStCshnFldTrgtPos_Val_read/1 -> Md62Calib/15(EepMd62ThdRwLtStCshnFldTrgtPos_Val_read)
  EepMd62ThdRwLtStFwdBkwdTrgtPos_Val_read/1 -> Md62Calib/16(EepMd62ThdRwLtStFwdBkwdTrgtPos_Val_read)
  EepMd62ThdRwRtStBkReclnTrgtPos_Val_read/1 -> Md62Calib/17(EepMd62ThdRwRtStBkReclnTrgtPos_Val_read)
  EepMd62ThdRwRtStCshnFldTrgtPos_Val_read/1 -> Md62Calib/18(EepMd62ThdRwRtStCshnFldTrgtPos_Val_read)
  EepMd62ThdRwRtStFwdBkwdTrgtPos_Val_read/1 -> Md62Calib/19(EepMd62ThdRwRtStFwdBkwdTrgtPos_Val_read)
  [MemReq] -> Md62Calib/21(MemReq)
  [CurrentPosArray] -> Md62Calib/20(CurrentPosArray)
  Md62Calib/9(Md62SecRwLtStLgrstUpwdDnwdTrgtPosCalib_TrgtPosArray_write) -> Md62SecRwLtStLgrstUpwdDnwdTrgtPosCalib_TrgtPosArray_write/1
  Md62Calib/8(Md62SecRwLtStLgrstInwdOtwdTrgtPosCalib_TrgtPosArray_write) -> Md62SecRwLtStLgrstInwdOtwdTrgtPosCalib_TrgtPosArray_write/1
  Md62Calib/10(Md62ThdRwLtStBkReclnUpwdDnwdTrgtPosCalib_TrgtPosArray_write) -> Md62ThdRwLtStBkReclnUpwdDnwdTrgtPosCalib_TrgtPosArray_write/1
  Md62Calib/7(Md62SecRwLtStFwdBkwdCalib_TrgtPosArray_write) -> Md62SecRwLtStFwdBkwdCalib_TrgtPosArray_write/1
  Md62Calib/11(Md62ThdRwLtStCshnFldUpwdDnwdTrgtPos_Val_write) -> Md62ThdRwLtStCshnFldUpwdDnwdTrgtPos_Val_write/1
  Md62Calib/6(Md62SecRwLtStCushFrntTrgtPosCalib_TrgtPosArray_write) -> Md62SecRwLtStCushFrntTrgtPosCalib_TrgtPosArray_write/1
  Md62Calib/12(Md62ThdRwLtStCshnFldUpwdDnwdTrgtPosCalib_TrgtPosArray_write) -> Md62ThdRwLtStCshnFldUpwdDnwdTrgtPosCalib_TrgtPosArray_write/1
  Md62Calib/5(Md62SecRwLtStBkReclnTrgtPosCalib_TrgtPosArray_write) -> Md62SecRwLtStBkReclnTrgtPosCalib_TrgtPosArray_write/1
  Md62Calib/13(Md62ThdRwLtStFrwdBkwdPosTrgtPosCalib_TrgtPosArray_write) -> Md62ThdRwLtStFrwdBkwdPosTrgtPosCalib_TrgtPosArray_write/1
  Md62Calib/4(Md62PassStFwdBkwdTrgtPosCalib_TrgtPosArray_write) -> Md62PassStFwdBkwdTrgtPosCalib_TrgtPosArray_write/1
  Md62Calib/14(Md62ThdRwRtStCshnFldUpwdDnwdTrgtPos_Val_write) -> Md62ThdRwRtStCshnFldUpwdDnwdTrgtPos_Val_write/1
  Md62Calib/3(Md62PassStCshnFldTrgtPosCalib_TrgtPosArray_write) -> Md62PassStCshnFldTrgtPosCalib_TrgtPosArray_write/1
  Md62Calib/2(Md62PassStBkReclnTrgtPosCalib_TrgtPosArray_write) -> Md62PassStBkReclnTrgtPosCalib_TrgtPosArray_write/1
  Md62Calib/1(Md62PassStBkReclnTrgtPos_Val_write) -> Md62PassStBkReclnTrgtPos_Val_write/1
  Md61Calib/15(Md61SecRwRtStBkReclnTrgtPosCalib_TrgtPosArray_write) -> Md61SecRwRtStBkReclnTrgtPosCalib_TrgtPosArray_write/1
  Md61Calib/16(Md61SecRwRtStCushFrntTrgtPosCalib_TrgtPosArray_write) -> Md61SecRwRtStCushFrntTrgtPosCalib_TrgtPosArray_write/1
  Md61Calib/17(Md61SecRwRtStFwdBkwdCalib_TrgtPosArray_write) -> Md61SecRwRtStFwdBkwdCalib_TrgtPosArray_write/1
  Md61Calib/18(Md61SecRwRtStLgrstInwdOtwdTrgtPosCalib_TrgtPosArray_write) -> Md61SecRwRtStLgrstInwdOtwdTrgtPosCalib_TrgtPosArray_write/1
  Md61Calib/19(Md61SecRwRtStLgrstUpwdDnwdTrgtPosCalib_TrgtPosArray_write) -> Md61SecRwRtStLgrstUpwdDnwdTrgtPosCalib_TrgtPosArray_write/1
  Md61Calib/20(Md61ThdRwRtStBkReclnUpwdDnwdTrgtPosCalib_TrgtPosArray_write) -> Md61ThdRwRtStBkReclnUpwdDnwdTrgtPosCalib_TrgtPosArray_write/1
  Md61Calib/21(Md61ThdRwRtStCshnFldUpwdDnwdTrgtPosCalib_TrgtPosArray_write) -> Md61ThdRwRtStCshnFldUpwdDnwdTrgtPosCalib_TrgtPosArray_write/1
  Md61Calib/22(Md61ThdRwRtStFrwdBkwdPosTrgtPosCalib_TrgtPosArray_write) -> Md61ThdRwRtStFrwdBkwdPosTrgtPosCalib_TrgtPosArray_write/1
  Md62Calib/15(Md62SecRwRtStBkReclnTrgtPosCalib_TrgtPosArray_write) -> Md62SecRwRtStBkReclnTrgtPosCalib_TrgtPosArray_write/1
  Md62Calib/16(Md62SecRwRtStCushFrntTrgtPosCalib_TrgtPosArray_write) -> Md62SecRwRtStCushFrntTrgtPosCalib_TrgtPosArray_write/1
  Md62Calib/17(Md62SecRwRtStFwdBkwdCalib_TrgtPosArray_write) -> Md62SecRwRtStFwdBkwdCalib_TrgtPosArray_write/1
  Md62Calib/18(Md62SecRwRtStLgrstInwdOtwdTrgtPosCalib_TrgtPosArray_write) -> Md62SecRwRtStLgrstInwdOtwdTrgtPosCalib_TrgtPosArray_write/1
  Md62Calib/19(Md62SecRwRtStLgrstUpwdDnwdTrgtPosCalib_TrgtPosArray_write) -> Md62SecRwRtStLgrstUpwdDnwdTrgtPosCalib_TrgtPosArray_write/1
  Md62Calib/20(Md62ThdRwRtStBkReclnUpwdDnwdTrgtPosCalib_TrgtPosArray_write) -> Md62ThdRwRtStBkReclnUpwdDnwdTrgtPosCalib_TrgtPosArray_write/1
  Md62Calib/21(Md62ThdRwRtStCshnFldUpwdDnwdTrgtPosCalib_TrgtPosArray_write) -> Md62ThdRwRtStCshnFldUpwdDnwdTrgtPosCalib_TrgtPosArray_write/1
  Md62Calib/22(Md62ThdRwRtStFrwdBkwdPosTrgtPosCalib_TrgtPosArray_write) -> Md62ThdRwRtStFrwdBkwdPosTrgtPosCalib_TrgtPosArray_write/1
  [ThdRwLtStCshnFldUpwdDnwdMovConfig] -> Md61Calib/22(ThdRwLtStCshnFldUpwdDnwdMovConfig)
  [ThdRwRtStCshnFldUpwdDnwdMovConfig] -> Md61Calib/23(ThdRwRtStCshnFldUpwdDnwdMovConfig)
  KeSMSwSeatBkLimitPos_Val/1 -> [KeSMSwSeatBkLimitPos], Md61Calib/24(KeSMSwSeatBkLimitPos_Val)
  KeSMSwSeatBkLimitPosDelt_Val/1 -> [KeSMSwSeatBkLimitPosDelt], Md61Calib/25(KeSMSwSeatBkLimitPosDelt_Val)
  [KeSMSwSeatBkLimitPos] -> Md62Calib/24(KeSMSwSeatBkLimitPos_Val)
  [KeSMSwSeatBkLimitPosDelt] -> Md62Calib/25(KeSMSwSeatBkLimitPosDelt_Val)
  [ThdRwRtStCshnFldUpwdDnwdMovConfig] -> Md62Calib/23(ThdRwRtStCshnFldUpwdDnwdMovConfig)
  [ThdRwLtStCshnFldUpwdDnwdMovConfig] -> Md62Calib/22(ThdRwLtStCshnFldUpwdDnwdMovConfig)
  Md62Calib/23(Md62PassStNeedFldOpn_Val_write) -> Md62PassStNeedFldOpn_Val_write/1
  Md62Calib/24(Md62PassStTrgtIsFld_Val_write) -> Md62PassStTrgtIsFld_Val_write/1
  Md62Calib/25(Md62ThdRwLtStNeedFldOpn_Val_write) -> Md62ThdRwLtStNeedFldOpn_Val_write/1
  Md62Calib/26(Md62ThdRwLtStTrgtIsFld_Val_write) -> Md62ThdRwLtStTrgtIsFld_Val_write/1
  Md62Calib/27(Md62ThdRwRtStNeedFldOpn_Val_write) -> Md62ThdRwRtStNeedFldOpn_Val_write/1
  Md62Calib/28(Md62ThdRwRtStTrgtIsFld_Val_write) -> Md62ThdRwRtStTrgtIsFld_Val_write/1
  Md61Calib/27(Md61ThdRwRtStNeedFldOpn_Val_write) -> Md61ThdRwRtStNeedFldOpn_Val_write/1
  Md61Calib/26(Md61ThdRwLtStTrgtIsFld_Val_write) -> Md61ThdRwLtStTrgtIsFld_Val_write/1
  Md61Calib/28(Md61ThdRwRtStTrgtIsFld_Val_write) -> Md61ThdRwRtStTrgtIsFld_Val_write/1
  Md61Calib/25(Md61ThdRwLtStNeedFldOpn_Val_write) -> Md61ThdRwLtStNeedFldOpn_Val_write/1
  Md61Calib/24(Md61PassStTrgtIsFld_Val_write) -> Md61PassStTrgtIsFld_Val_write/1
  Md61Calib/23(Md61PassStNeedFldOpn_Val_write) -> Md61PassStNeedFldOpn_Val_write/1
  modestate32_Val_read/1 -> [modestate32], Md61Calib/31(modestate32_Val_read)
  Md61Calib/30(EepMd61PassStCshnFldTrgtPos_S_Val_write) -> EepMd61PassStCshnFldTrgtPos_S_Val_write/1
  Md61Calib/29(EepMd61PassStBkReclnTrgtPos_S_Val_write) -> EepMd61PassStBkReclnTrgtPos_S_Val_write/1
  Md61Calib/31(EepMd61PassStFwdBkwdTrgtPos_S_Val_write) -> EepMd61PassStFwdBkwdTrgtPos_S_Val_write/1
  Md61Calib/32(EepMd61SecRwLtStBkReclnTrgtPos_S_Val_write) -> EepMd61SecRwLtStBkReclnTrgtPos_S_Val_write/1
  Md61Calib/33(EepMd61SecRwLtStCushFrntTrgtPos_S_Val_write) -> EepMd61SecRwLtStCushFrntTrgtPos_S_Val_write/1
  Md61Calib/34(EepMd61SecRwLtStFwdBkwdTrgtPos_S_Val_write) -> EepMd61SecRwLtStFwdBkwdTrgtPos_S_Val_write/1
  Md61Calib/35(EepMd61SecRwLtStLgrstInwdOtwdTrgtPos_S_Val_write) -> EepMd61SecRwLtStLgrstInwdOtwdTrgtPos_S_Val_write/1
  Md61Calib/36(EepMd61SecRwLtStLgrstUpwdDnwdTrgtPos_S_Val_write) -> EepMd61SecRwLtStLgrstUpwdDnwdTrgtPos_S_Val_write/1
  Md61Calib/37(EepMd61SecRwRtStBkReclnTrgtPos_S_Val_write) -> EepMd61SecRwRtStBkReclnTrgtPos_S_Val_write/1
  Md61Calib/38(EepMd61SecRwRtStCushFrntTrgtPos_S_Val_write) -> EepMd61SecRwRtStCushFrntTrgtPos_S_Val_write/1
  Md61Calib/39(EepMd61SecRwRtStFwdBkwdTrgtPos_S_Val_write) -> EepMd61SecRwRtStFwdBkwdTrgtPos_S_Val_write/1
  Md61Calib/40(EepMd61SecRwRtStLgrstInwdOtwdTrgtPos_S_Val_write) -> EepMd61SecRwRtStLgrstInwdOtwdTrgtPos_S_Val_write/1
  Md61Calib/41(EepMd61SecRwRtStLgrstUpwdDnwdTrgtPos_S_Val_write) -> EepMd61SecRwRtStLgrstUpwdDnwdTrgtPos_S_Val_write/1
  Md61Calib/42(EepMd61ThdRwLtStBkReclnTrgtPos_S_Val_write) -> EepMd61ThdRwLtStBkReclnTrgtPos_S_Val_write/1
  Md61Calib/43(EepMd61ThdRwLtStCshnFldTrgtPos_S_Val_write) -> EepMd61ThdRwLtStCshnFldTrgtPos_S_Val_write/1
  Md61Calib/44(EepMd61ThdRwLtStFwdBkwdTrgtPos_S_Val_write) -> EepMd61ThdRwLtStFwdBkwdTrgtPos_S_Val_write/1
  Md61Calib/45(EepMd61ThdRwRtStBkReclnTrgtPos_S_Val_write) -> EepMd61ThdRwRtStBkReclnTrgtPos_S_Val_write/1
  Md61Calib/46(EepMd61ThdRwRtStCshnFldTrgtPos_S_Val_write) -> EepMd61ThdRwRtStCshnFldTrgtPos_S_Val_write/1
  Md61Calib/47(EepMd61ThdRwRtStFwdBkwdTrgtPos_S_Val_write) -> EepMd61ThdRwRtStFwdBkwdTrgtPos_S_Val_write/1
  Md62Calib/29(EepMd62PassStBkReclnTrgtPos_S_Val_write) -> EepMd62PassStBkReclnTrgtPos_S_Val_write/1
  Md62Calib/30(EepMd62PassStCshnFldTrgtPos_S_Val_write) -> EepMd62PassStCshnFldTrgtPos_S_Val_write/1
  Md62Calib/31(EepMd62PassStFwdBkwdTrgtPos_S_Val_write) -> EepMd62PassStFwdBkwdTrgtPos_S_Val_write/1
  Md62Calib/32(EepMd62SecRwLtStBkReclnTrgtPos_S_Val_write) -> EepMd62SecRwLtStBkReclnTrgtPos_S_Val_write/1
  Md62Calib/33(EepMd62SecRwLtStCushFrntTrgtPos_S_Val_write) -> EepMd62SecRwLtStCushFrntTrgtPos_S_Val_write/1
  Md62Calib/34(EepMd62SecRwLtStFwdBkwdTrgtPos_S_Val_write) -> EepMd62SecRwLtStFwdBkwdTrgtPos_S_Val_write/1
  Md62Calib/35(EepMd62SecRwLtStLgrstInwdOtwdTrgtPos_S_Val_write) -> EepMd62SecRwLtStLgrstInwdOtwdTrgtPos_S_Val_write/1
  Md62Calib/36(EepMd62SecRwLtStLgrstUpwdDnwdTrgtPos_S_Val_write) -> EepMd62SecRwLtStLgrstUpwdDnwdTrgtPos_S_Val_write/1
  Md62Calib/37(EepMd62SecRwRtStBkReclnTrgtPos_S_Val_write) -> EepMd62SecRwRtStBkReclnTrgtPos_S_Val_write/1
  Md62Calib/38(EepMd62SecRwRtStCushFrntTrgtPos_S_Val_write) -> EepMd62SecRwRtStCushFrntTrgtPos_S_Val_write/1
  Md62Calib/39(EepMd62SecRwRtStFwdBkwdTrgtPos_S_Val_write) -> EepMd62SecRwRtStFwdBkwdTrgtPos_S_Val_write/1
  Md62Calib/40(EepMd62SecRwRtStLgrstInwdOtwdTrgtPos_S_Val_write) -> EepMd62SecRwRtStLgrstInwdOtwdTrgtPos_S_Val_write/1
  Md62Calib/41(EepMd62SecRwRtStLgrstUpwdDnwdTrgtPos_S_Val_write) -> EepMd62SecRwRtStLgrstUpwdDnwdTrgtPos_S_Val_write/1
  Md62Calib/42(EepMd62ThdRwLtStBkReclnTrgtPos_S_Val_write) -> EepMd62ThdRwLtStBkReclnTrgtPos_S_Val_write/1
  Md62Calib/43(EepMd62ThdRwLtStCshnFldTrgtPos_S_Val_write) -> EepMd62ThdRwLtStCshnFldTrgtPos_S_Val_write/1
  Md62Calib/44(EepMd62ThdRwLtStFwdBkwdTrgtPos_S_Val_write) -> EepMd62ThdRwLtStFwdBkwdTrgtPos_S_Val_write/1
  Md62Calib/45(EepMd62ThdRwRtStBkReclnTrgtPos_S_Val_write) -> EepMd62ThdRwRtStBkReclnTrgtPos_S_Val_write/1
  Md62Calib/46(EepMd62ThdRwRtStCshnFldTrgtPos_S_Val_write) -> EepMd62ThdRwRtStCshnFldTrgtPos_S_Val_write/1
  Md62Calib/47(EepMd62ThdRwRtStFwdBkwdTrgtPos_S_Val_write) -> EepMd62ThdRwRtStFwdBkwdTrgtPos_S_Val_write/1
  Md61Calib/48(Md61MemReq_Val_write) -> Md61MemReq_Val_write/1
  Md62Calib/48(Md62MemReq_Val_write) -> Md62MemReq_Val_write/1
  Md61Calib/49(Md61NotMem_Val_write) -> Md61NotMem_Val_write/1
  Md62Calib/49(Md62NotMem_Val_write) -> Md62NotMem_Val_write/1
  [IfVeSMSuSecRwRtStBkReclnUpwdDnwdPos] -> Md61Calib/27(IfVeSMSuSecRwRtStBkReclnUpwdDnwdPos)
  [IfVeSMSuSecRwLtStFrwdBkwdPos] -> Md61Calib/28(IfVeSMSuSecRwLtStFrwdBkwdPos)
  [IfVeSMSuSecRwLtStBkReclnUpwdDnwdPos] -> Md61Calib/29(IfVeSMSuSecRwLtStBkReclnUpwdDnwdPos)
  [IfVeSMSuSecRwRtStFrwdBkwdPos] -> Md61Calib/30(IfVeSMSuSecRwRtStFrwdBkwdPos)
  [IfVeSMSuSecRwRtStBkReclnUpwdDnwdPos] -> Md62Calib/26(IfVeSMSuSecRwRtStBkReclnUpwdDnwdPos)
  [IfVeSMSuSecRwLtStFrwdBkwdPos] -> Md62Calib/27(IfVeSMSuSecRwLtStFrwdBkwdPos)
  [IfVeSMSuSecRwLtStBkReclnUpwdDnwdPos] -> Md62Calib/28(IfVeSMSuSecRwLtStBkReclnUpwdDnwdPos)
  [IfVeSMSuSecRwRtStFrwdBkwdPos] -> Md62Calib/29(IfVeSMSuSecRwRtStFrwdBkwdPos)
  [modestate32] -> Md62Calib/30(modestate32_Val_read)
  [IfVeSMSuPassStBkReclnUpwdDnwdPosV] -> Md61Calib/26(IfVeSMSuPassStBkReclnUpwdDnwdPosV_Val_read)
  [IfVeSMSuPassStBkReclnUpwdDnwdPosV] -> Md62Calib/31(IfVeSMSuPassStBkReclnUpwdDnwdPosV)
